simulink model "MPPT_sim"  (R2024b)
settings: Solver=VariableStepAuto  StartTime=0.0  StopTime=2  RelTol=1e-3
undefined symbols (not defined in the file): Ion, Lithium
libraries: spsSeriesRLCBranchLib x3, simulink x2, spsBatteryLib x1, spsDiodeLib x1, spsIGBTLib x1, eePwmGenerator x1, spsPVArrayLib x1, spspowerguiLib x1
settings Model: Creator=himan  LastModifiedBy=himan
settings ModelReferenceCC: EnableRefExpFcnMdlSchedulingChecks=on
settings RTWCC: GPUComputeCapability=3.5

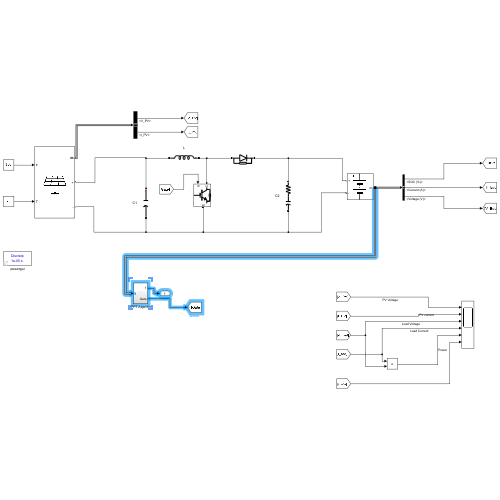
[thumbnail: Simulink's stored preview of the top-level diagram]
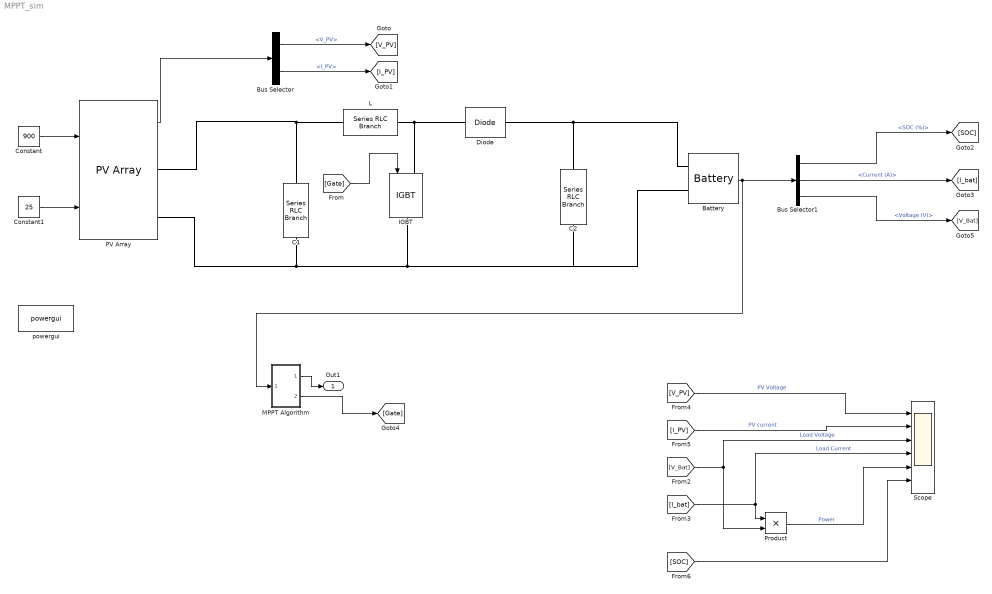
== system MPPT_sim ==
  Battery : spsBatteryLib/Battery  BatType=Lithium-Ion  NomV=48  NomQ=100  SOC=40  Batt_Tr=0.250  PresetModel=on  MaxQ=100  MinV=36  FullV=55.8714  Dis_rate=43.4783  R=0.0048  Normal_OP=90.4348  expZone="[51.8585      4.91304]"
  Bus Selector : BusSelector  OutputSignals=V_PV,I_PV
  Bus Selector1 : BusSelector  OutputSignals=SOC (%),Current (A),Voltage (V)
  C1 : spsSeriesRLCBranchLib/Series RLC Branch  LConnTagsString=__new0  RConnTagsString=__new0  BranchType=C  Resistance=0  Inductance=0  SetiL0=off  InitialCurrent=0  Capacitance=1e-3  Setx0=off  InitialVoltage=0  Measurements=None
  C2 : spsSeriesRLCBranchLib/Series RLC Branch  LConnTagsString=__new0  RConnTagsString=__new0  BranchType=RC  Resistance=1e-4  Inductance=0  SetiL0=off  InitialCurrent=0  Capacitance=10e-6  Setx0=off  InitialVoltage=0  Measurements=None
  Constant : Constant  Value=900
  Constant1 : Constant  Value=25
  Diode : spsDiodeLib/Diode  Ron=0.001  Lon=0  Vf=0.8  IC=0  UseSnubber=0  Rs=500  Cs=250e-9  Measurements=off
  IGBT : spsIGBTLib/IGBT  Ron=0.001  Lon=0  Vf=1  Tf=1e-6  Tt=2e-6  IC=0  Rs=1e5  Cs=inf  Measurements=off
  L : spsSeriesRLCBranchLib/Series RLC Branch  LConnTagsString=__new0  RConnTagsString=__new0  BranchType=L  Resistance=0  Inductance=1e-1  SetiL0=off  InitialCurrent=0  Capacitance=1e-6  Setx0=off  InitialVoltage=0  Measurements=None
  MPPT Algorithm : Subsystem
  PV Array : spsPVArrayLib/PV Array  Npar=1  Nser=1  PlotType=array @ 25 deg.C & specified irradiances  S_vec="[ 1000  800 ]"  Temp_C_vec="[ 45 25  ]"  ModuleName=User-defined  PlotWhenSelected=off  Pm=535.392  Ncell=144  Voc=49.4  Isc=13.56  Vm=41.6  Im=12.87  beta_Voc_pc=-0.27  alpha_Isc_pc=0.05  beta_Voc=-0.13338  alpha_Isc=0.00678  IL=13.5812  I0=1.2378e-11  nI=0.48183  Rsh=307.5281  Rs=0.17005  RobustModel=off  RobustCellTemperature=313.3991  BAL=on  Tc=1e-6  Tfilter=5e-5
  Product : Product
  Scope : Scope  NumInputPorts=6
  powergui : spspowerguiLib/powergui  Priority=1  SimulationMode=Discrete  SampleTime=1e-5  frequency=60  Iterations=50  frequencyindice=0  Pbase=100e6  ErrMax=1e-4  UnitsV=kV  UnitsW=MW  buscounter=0  FunctionMessages=off  echomessages=off  EnableUseOfTLC=off  CurrentSourceSwitches=off  DisableSnubberDevices=off  DisableRonSwitches=off  DisableVfSwitches=off  DisplayEquations=off  AutomaticDiscreteSolvers=off  SolverType=Tustin/Backward Euler (TBE)  Interpol=off  ExternalGateDelay=off  methode=off  Ts=100  x0status=blocks  SPID=on  SwTol=0  HookPort=off  NonlinearTolerance=1e-4  nMaxIteration=100  ContinueOnMaxIteration=off  RestoreLinks=warning  ResistiveCurrentMeasurement=off  Frange=[0:2:500]  Ylog=off  Xlog=on  ShowGrid=off  save=off  variable=ZData  structure=0  ZoomFFT=off  StartTime=0.0  cycles=1  DisplayStyle=1  fundamental=60  FreqAxis=off  MaxFrequency=1000  frequencyindicesteady=1  RmsSteady=1  display=off
  Out1 : Outport
  wires:
  Constant/1 -> PV Array/1
  Constant1/1 -> PV Array/2
  PV Array/1 -> Bus Selector/1
  Bus Selector/1 -> [V_PV]  "<V_PV>"
  Bus Selector/2 -> [I_PV]  "<I_PV>"
  MPPT Algorithm/1(Out1) -> Out1/1
  [Gate] -> IGBT/1
  Bus Selector1/2 -> [I_bat]  "<Current (A)>"
  Bus Selector1/1 -> [SOC]  "<SOC (%)>"
  Battery/1 -> Bus Selector1/1, MPPT Algorithm/1(In1)
  Bus Selector1/3 -> [V_Bat]  "<Voltage (V)>"
  [I_PV] -> Scope/2  "PV current"
  [V_PV] -> Scope/1  "PV Voltage"
  [SOC] -> Scope/6
  Product/1 -> Scope/5  "Power"
  [V_Bat] -> Product/2, Scope/3  "Load Voltage"
  [I_bat] -> Product/1, Scope/4  "Load Current"
  MPPT Algorithm/2(Gate) -> [Gate]
  connections:
  C1/LConn1 -- PV Array/RConn1 -- L/RConn1
  PV Array/RConn2 -- C2/RConn1 -- Battery/LConn2 -- IGBT/RConn1 -- C1/RConn1
  L/LConn1 -- Diode/LConn1 -- IGBT/LConn1
  Diode/RConn1 -- Battery/LConn1 -- C2/LConn1

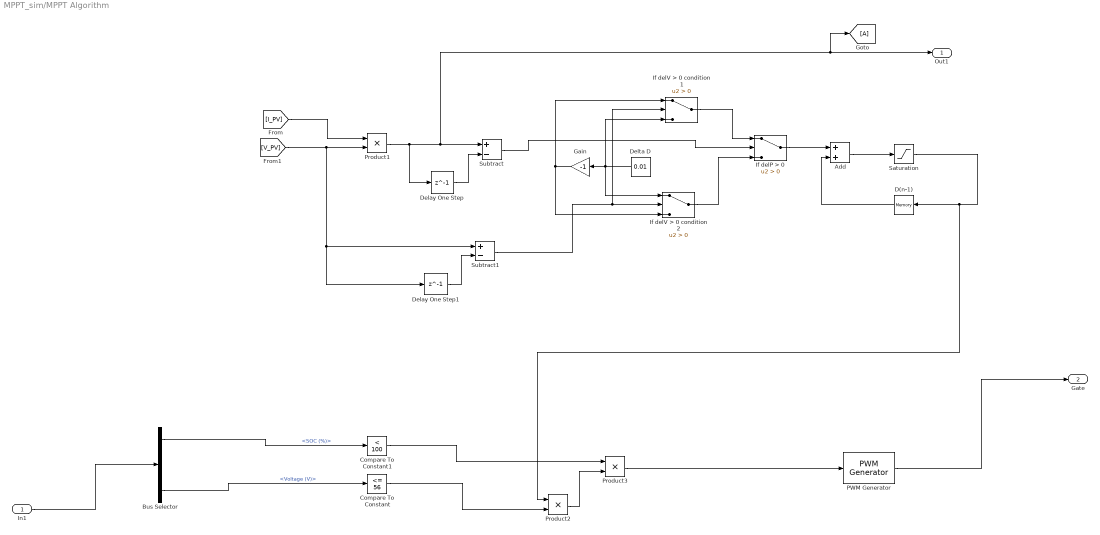
== system MPPT_sim/MPPT Algorithm ==
  In1 : Inport
  Add : Sum
  Bus Selector : BusSelector  OutputSignals=SOC (%),Current (A),Voltage (V)
  Compare To Constant : simulink/Logic and Bit Operations/Compare To Constant  relop=<=  const=56  OutDataTypeStr=boolean
  Compare To Constant1 : simulink/Logic and Bit Operations/Compare To Constant  relop=<  const=100  OutDataTypeStr=boolean
  D(n-1) : Memory  InheritSampleTime=on
  Delay One Step : Delay  DelayLength=1
  Delay One Step1 : Delay  DelayLength=1
  Delta D : Constant  Value=0.01
  Gain : Gain  Gain=-1
  Goto : Goto
  "If delP > 0 " : Switch  Criteria=u2 > Threshold  SaturateOnIntegerOverflow=off  InputSameDT=off
  If delV > 0 condition 1 : Switch  Criteria=u2 > Threshold  SaturateOnIntegerOverflow=off  InputSameDT=off
  "If delV > 0 condition 2 " : Switch  Criteria=u2 > Threshold  SaturateOnIntegerOverflow=off  InputSameDT=off
  PWM Generator : eePwmGenerator/PWM Generator  CarrCount=Up  Tper=0.0001  Tdelay=0  Ts=1e-6
  Product1 : Product
  Product2 : Product
  Product3 : Product
  Saturation : Saturate  UpperLimit=1  LowerLimit=0
  Subtract : Sum  Inputs=+-
  Subtract1 : Sum  Inputs=+-
  Out1 : Outport
  Gate : Outport  Port=2
  wires:
  [V_PV] -> Delay One Step1/1, Subtract1/1, Product1/2
  Add/1 -> Saturation/1
  Delta D/1 -> "If delV > 0 condition 2 "/1, If delV > 0 condition 1/3, Gain/1
  Gain/1 -> "If delV > 0 condition 2 "/3, If delV > 0 condition 1/1
  Saturation/1 -> Product2/1, D(n-1)/1
  Subtract/1 -> "If delP > 0 "/2
  Subtract1/1 -> If delV > 0 condition 1/2, "If delV > 0 condition 2 "/2
  "If delP > 0 "/1 -> Add/1
  "If delV > 0 condition 2 "/1 -> "If delP > 0 "/3
  [I_PV] -> Product1/1
  Product1/1 -> Goto/1, Out1/1, Subtract/1, Delay One Step/1
  Delay One Step1/1 -> Subtract1/2
  D(n-1)/1 -> Add/2
  If delV > 0 condition 1/1 -> "If delP > 0 "/1
  Delay One Step/1 -> Subtract/2
  PWM Generator/1 -> Gate/1
  In1/1 -> Bus Selector/1
  Product2/1 -> Product3/2
  Product3/1 -> PWM Generator/1
  Compare To Constant1/1 -> Product3/1
  Compare To Constant/1 -> Product2/2
  Bus Selector/1 -> Compare To Constant1/1  "<SOC (%)>"
  Bus Selector/3 -> Compare To Constant/1  "<Voltage (V)>"
